simulink model "ConsignasPrueba"  (R2023b)
settings: Solver=VariableStepAuto  StartTime=0.0  StopTime=15  MaxStep=1e-3  RelTol=1e-3
settings Model: Creator=Home  LastModifiedBy=Home

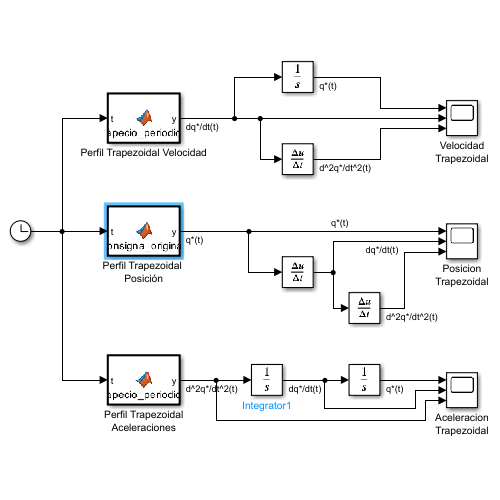
[thumbnail: Simulink's stored preview of the top-level diagram]
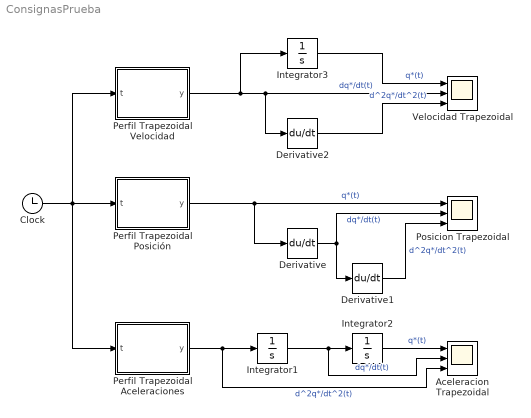
== system ConsignasPrueba ==
  Aceleracion Trapezoidal : Scope  NumInputPorts=3
  Clock : Clock
  Derivative : Derivative
  Derivative1 : Derivative
  Derivative2 : Derivative
  Integrator1 : Integrator
  Integrator2 : Integrator
  Integrator3 : Integrator
  Perfil Trapezoidal Aceleraciones : MATLAB Function  TreatAsAtomicUnit=on
  Perfil Trapezoidal Posición : MATLAB Function  TreatAsAtomicUnit=on
  Perfil Trapezoidal Velocidad : MATLAB Function  TreatAsAtomicUnit=on
  Posicion Trapezoidal : Scope  NumInputPorts=3
  Velocidad Trapezoidal : Scope  NumInputPorts=3
  wires:
  Perfil Trapezoidal Posición/1(y) -> Derivative/1, Posicion Trapezoidal/1  "q*(t)"
  Clock/1 -> Perfil Trapezoidal Velocidad/1(t), Perfil Trapezoidal Aceleraciones/1(t), Perfil Trapezoidal Posición/1(t)
  Derivative/1 -> Derivative1/1, Posicion Trapezoidal/2  "dq*/dt(t)"
  Perfil Trapezoidal Aceleraciones/1(y) -> Aceleracion Trapezoidal/3, Integrator1/1  "d^2q*/dt^2(t)"
  Integrator1/1 -> Aceleracion Trapezoidal/2, Integrator2/1  "dq*/dt(t)"
  Integrator2/1 -> Aceleracion Trapezoidal/1  "q*(t)"
  Derivative1/1 -> Posicion Trapezoidal/3  "d^2q*/dt^2(t)"
  Perfil Trapezoidal Velocidad/1(y) -> Integrator3/1, Derivative2/1, Velocidad Trapezoidal/2  "dq*/dt(t)"
  Integrator3/1 -> Velocidad Trapezoidal/1  "q*(t)"
  Derivative2/1 -> Velocidad Trapezoidal/3  "d^2q*/dt^2(t)"

== matlab function ConsignasPrueba/Perfil Trapezoidal Posición ==
  data: t input; y output
function y = consigna_original(t)
    % Parámetros
    T = 15;              % Periodo total
    ramp_time = 0.5;     % Duración de la rampa (en segundos)
    amplitude = 2 * pi; % Amplitud del trapecio


    % Calcular el tiempo dentro del período
    t_mod = mod(t, T);

    % Inicializar salida
    y = 0;

    if t_mod >= 0 && t_mod < T/3
        y = amplitude * t_mod/(T/3);
    end
    if t_mod >= T/3 && t_mod < 2*T/3
        y = amplitude;
    end
    if t_mod >= 2*T/3 && t_mod < T
        y = amplitude * (1 - (t_mod - 2*T/3)/(T/3));
    end
end

== matlab function ConsignasPrueba/Perfil Trapezoidal Velocidad ==
  data: t input; y output
function y = trapecio_periodico(t)
    % Parámetros
    T = 15;              % Periodo total
    ramp_time = 0.5;     % Duración de la rampa (en segundos)
    amplitude = 2 * pi / 5; % Amplitud del trapecio
    
    %% Calculo de parámetros
    tr1 = 0.25;
    h1 = 4*pi/(10-2*tr1);

    % Calcular el tiempo dentro del período
    t_mod = mod(t, T);

    % Inicializar salida
    y = 0;
    
    %% Fase 1: Primer trapecio
    if t_mod >= 0 && t_mod < T/3
        if t_mod < tr1
            y = h1 * t_mod / tr1;
        elseif t_mod >= tr1 && t_mod < T/3 - tr1
            y = h1;
        elseif t_mod >= T/3 - tr1 && t_mod < T/3
            y = h1 * (1 - (t_mod - (T/3 - tr1))/ tr1);
        end
    end

    %% Fase 2: Segundo trapecio
    if t_mod >= 2*T/3 && t_mod < T
        if t_mod < 2*T/3 + tr1
            y = - h1 * (t_mod - (2*T/3))/ tr1;
        elseif t_mod >= 2*T/3 + tr1 && t_mod < T - tr1
            y = - h1;
        elseif t_mod >= T - tr1
            y = h1 * (-1 + (t_mod - (T - tr1))/ tr1);
        end
    end

end

== matlab function ConsignasPrueba/Perfil Trapezoidal Aceleraciones ==
  data: t input; y output
function y = trapecio_periodico(t)
    % Parámetros
    T = 15;              % Periodo total
    ramp_time = 0.5;     % Duración de la rampa (en segundos)
    amplitude = 2 * pi / 5; % Amplitud del trapecio
    
    %% Calculo de parámetros
    tr1 = 0.25;
    tr2 = tr1/5;
    h1 = 4*pi/(10-2*tr1);
    h2 = 2*h1/(2*tr1-2*tr2);

    % Calcular el tiempo dentro del período
    t_mod = mod(t, T);

    % Inicializar salida
    y = 0;

    %% Fase 1: Primer trapecio (0 <= t_mod < tr1)
    if t_mod >= 0 && t_mod < tr1
        if t_mod < tr2
            % Rampa ascendente (inicio)
            y = h2 * (t_mod / tr2);
        elseif t_mod >= tr2 && t_mod <= (tr1 - tr2)
            % Parte constante (plataforma)
            y = h2;
        elseif t_mod > (tr1 - tr2) && t_mod <= tr1
            % Rampa descendente (fin)
            y = h2 * (1 - (t_mod - (tr1 - tr2)) / tr2);
        end
    end

    %% Fase 2: Segundo trapecio (5 - tr1 <= t_mod < 5)
    if t_mod >= 5-tr1 && t_mod < 5
        if t_mod < (5-tr1+tr2)
            % Rampa descendente (inicio)
            y = -h2 * ((t_mod - (5-tr1)) / tr2);
        elseif t_mod >= (5-tr1+tr2) && t_mod <= (5-tr2)
            % Parte constante (plataforma)
            y = -h2;
        elseif t_mod > (5-tr2) && t_mod < 5
            % Rampa ascendente (fin)
            y = -h2 * (1 - (t_mod - (5-tr2)) / tr2);
        end
    end

    %% Fase 3: Tercer trapecio (10 <= t_mod < 10 + tr1)
    if t_mod >= 10 && t_mod < 10 + tr1
        if t_mod < (10 + tr2)
            % Rampa descendente (inicio)
            y = -h2 * ((t_mod - (10)) / tr2);
        elseif t_mod >= (10 + tr2) && t_mod <= (10 + tr1 - tr2)
            % Parte constante (plataforma)
            y = -h2;
        elseif t_mod > (10 + tr1 - tr2) && t_mod < 10 + tr1
            % Rampa ascendente (fin)
            y = -h2 * (1 - (t_mod - (10 + tr1 - tr2)) / tr2);
        end
    end

    %% Fase 4: Cuarto trapecio (15 - tr1 <= t_mod < 15)
    if t_mod >= 15 - tr1 && t_mod < 15
        if t_mod < 15 - tr1 +tr2
            % Rampa ascendente (inicio)
            y = h2 * ((t_mod - (15 - tr1))/ tr2);
        elseif t_mod >= 15 - tr1 + tr2 && t_mod <= (15-tr2)
            % Parte constante (plataforma)
            y = h2;
        elseif t_mod > (15 - tr2) && t_mod <= 15
            % Rampa descendente (fin)
            y = h2 * (1 - (t_mod - (15 - tr2)) / tr2);
        end
    end
end
